simulink model "afe_dq_inv_3L_psm"  (R2025a)
settings: Solver=ode1be  StartTime=0.0  StopTime=simlength  FixedStep=tc  MaxStep=tc
undefined symbols (not defined in the file): Adrso, Amplitude_U, Amplitude_V, Amplitude_W, b, Crso, CTRPIFF_CLIP_RELEASE, dead_time_AFE, dead_time_INV, deepNEGeta, deepNEGxi, deepPOSxi, emf_fb_p, emf_fb_p_ccaller_1, emf_fb_p_ccaller_2, emf_p, emf_p_ccaller_1, emf_p_ccaller_2, end_time_LVRT, fPWM_AFE, fPWM_INV, g0_500Hz, g1_500Hz, ibez, id_lim, Igrid_phase_normalization_factor, iq_lim, ixi_pos_ref_lim, Jm, kg, ki_afe, ki_i, ki_rc_grid, ki_vs, ki_w, kp_afe, kp_i, kp_rc_grid, kp_vs, kp_w, kw, Ld_norm, Ldrso, Lq_norm, Ls_norm, magnitude, motorc_m_scale, n1, n10, omega_bez, omega_grid_emulator_nom, omega_grid_nom, omega_m_bez, omega_m_sim, Phase_shift, pll_i1, pll_i1_ddsrt, pll_p, pll_p_ddsrt, pll_p_frt ... (+28)
libraries: fl_lib x159, nesl_utility x86, cstblocks x14, single_phase_transformer_lib x3, threephase_inductor_lib x2, simulink x2, flexshaft_lib x1, pmsm_uvw_with_harmonics_lib x1
(part 8 of 9)

== system afe_dq_inv_3L_psm/afe_dq_inv_psm_mod1/afe_control/grid_voltage_phase_lock_loops/DQ-PLL/pll_stageA/mormalization_and_transformation ==
  ug_a : Inport
  ug_b : Inport  Port=2
  ug_c : Inport  Port=3
  Gain1 : Gain  Gain=1/Vgrid_phase_normalization_factor
  Gain2 : Gain  Gain=1/Vgrid_phase_normalization_factor
  Gain3 : Gain  Gain=1/Vgrid_phase_normalization_factor
  Mux : Mux  Inputs=3
  Quantizer1 : Quantizer  QuantizationInterval=adc_quantization
  Quantizer2 : Quantizer  QuantizationInterval=adc_quantization
  Quantizer4 : Quantizer  QuantizationInterval=adc_quantization
  Unit Delay : UnitDelay  SampleTime=ts_afe  HasFrameUpgradeWarning=on
  Unit Delay1 : UnitDelay  SampleTime=ts_afe  HasFrameUpgradeWarning=on
  Unit Delay2 : UnitDelay  SampleTime=ts_afe  HasFrameUpgradeWarning=on
  Zero-Order Hold1 : ZeroOrderHold  SampleTime=-1
  Zero-Order Hold3 : ZeroOrderHold  SampleTime=-1
  Zero-Order Hold4 : ZeroOrderHold  SampleTime=-1
  abc2alphabeta : MATLAB Function  TreatAsAtomicUnit=on  SystemSampleTime=ts_afe
  u_500Hz_flt : Subsystem
  u_500Hz_flt1 : Subsystem
  u_500Hz_flt2 : Subsystem
  ug_alpha : Outport  VectorParamsAs1DForOutWhenUnconnected=off
  ug_beta : Outport  Port=2  VectorParamsAs1DForOutWhenUnconnected=off
  tag scope: v_grid_ff_abc=global
  wires:
  abc2alphabeta/2(beta) -> ug_beta/1  "u_grid_beta"
  abc2alphabeta/1(alpha) -> ug_alpha/1  "u_grid_alpha"
  u_500Hz_flt1/1(output) -> Mux/2
  u_500Hz_flt2/1(output) -> Mux/3
  u_500Hz_flt/1(output) -> Mux/1
  Unit Delay/1 -> u_500Hz_flt2/1(input), abc2alphabeta/3(c)
  Unit Delay1/1 -> u_500Hz_flt1/1(input), abc2alphabeta/2(b)
  Mux/1 -> [v_grid_ff_abc]
  Unit Delay2/1 -> u_500Hz_flt/1(input), abc2alphabeta/1(a)
  Zero-Order Hold4/1 -> Unit Delay/1
  Gain1/1 -> Quantizer4/1
  Gain2/1 -> Quantizer1/1
  ug_a/1 -> Gain3/1
  Gain3/1 -> Quantizer2/1
  ug_c/1 -> Gain1/1
  Quantizer2/1 -> Zero-Order Hold1/1
  Zero-Order Hold3/1 -> Unit Delay1/1
  ug_b/1 -> Gain2/1
  Quantizer1/1 -> Zero-Order Hold3/1
  Quantizer4/1 -> Zero-Order Hold4/1
  Zero-Order Hold1/1 -> Unit Delay2/1

== system afe_dq_inv_3L_psm/afe_dq_inv_psm_mod1/afe_control/grid_voltage_phase_lock_loops/DQ-PLL/pll_stageA/sequences ==
  u_grid_alpha : Inport
  u_grid_beta : Inport  Port=2
  gamma_grid : Inport  Port=3
  alphabeta2xieta : Subsystem
  u_grid_pos_xi : Outport
  u_grid_pos_eta : Outport  Port=2
  wires:
  alphabeta2xieta/1(xi) -> u_grid_pos_xi/1  "u_grid_pos_xi"
  alphabeta2xieta/2(eta) -> u_grid_pos_eta/1  "u_grid_pos_eta"
  u_grid_alpha/1 -> alphabeta2xieta/1(alpha)  "u_grid_alpha"
  u_grid_beta/1 -> alphabeta2xieta/2(beta)  "u_grid_beta"
  gamma_grid/1 -> alphabeta2xieta/3(gamma)  "gamma_grid"

== system afe_dq_inv_3L_psm/afe_dq_inv_psm_mod1/afe_control/grid_voltage_phase_lock_loops/DQ-PLL/pll_stageB/double_integrator_observer ==
  theta : Inport
  Gain : Gain  Gain=Ldrso  Multiplication=Matrix(K*u)
  Gain1 : Gain  Gain=Adrso  Multiplication=Matrix(K*u)
  Gain2 : Gain  Gain=Crso  Multiplication=Matrix(K*u)
  Selector : Selector  InputPortWidth=2  IndexOptions=Index vector (dialog)  Indices=2  OutputSizes=1
  Sum : Sum  Inputs=-+|
  Sum1 : Sum  Inputs=|++
  Unit Delay : UnitDelay  SampleTime=ts_afe  HasFrameUpgradeWarning=on
  Zero-Order Hold : ZeroOrderHold  SampleTime=ts_afe
  bounder1 : MATLAB Function  TreatAsAtomicUnit=on  SystemSampleTime=ts_afe
  bounder2 : MATLAB Function  TreatAsAtomicUnit=on  SystemSampleTime=ts_afe
  omega_hat : Outport
  wires:
  Gain/1 -> Sum1/1
  Selector/1 -> omega_hat/1
  Gain2/1 -> bounder2/1(u)  "theta_hat"
  Gain1/1 -> Sum1/2
  Sum1/1 -> Unit Delay/1
  Sum/1 -> bounder1/1(u)  "e"
  Unit Delay/1 -> Gain1/1, Selector/1, Gain2/1
  theta/1 -> Zero-Order Hold/1  "theta"
  Zero-Order Hold/1 -> Sum/2  "theta_dsp"
  bounder1/1(y) -> Gain/1  "e_bounded"
  bounder2/1(y) -> Sum/1  "theta_hat_bounded"

== system afe_dq_inv_3L_psm/afe_dq_inv_psm_mod1/afe_control/grid_voltage_phase_lock_loops/DQ-PLL/pll_stageB/scheduled-p-gain ==
  In1 : Inport
  Switch : Switch  Criteria=u2 > Threshold  Threshold=0.5  SaturateOnIntegerOverflow=off  InputSameDT=off
  kp1 : Gain  Gain=pll_p  SaturateOnIntegerOverflow=on  OutDataTypeStr=Inherit: Same as input  ParamDataTypeStr=Inherit: Same as input
  kp3 : Gain  Gain=pll_p_frt  SaturateOnIntegerOverflow=on  OutDataTypeStr=Inherit: Same as input  ParamDataTypeStr=Inherit: Same as input
  Out2 : Outport
  wires:
  kp3/1 -> Switch/1
  kp1/1 -> Switch/3
  [frt_active] -> Switch/2
  In1/1 -> kp1/1, kp3/1
  Switch/1 -> Out2/1

== system afe_dq_inv_3L_psm/afe_dq_inv_psm_mod1/inverter/inverter/sv_pwm/modulator1/PWM generator u ==
  m : Inport
  phase : Inport  Port=2
  Bus Creator : BusCreator  Inputs=4
  Constant : Constant
  Gain : Gain  Gain=2
  Sum : Sum  Inputs=|+-
  carry_p : Subsystem
  modulator_n1 : Subsystem
  modulator_p1 : Subsystem
  mu : Outport
  wires:
  phase/1 -> carry_p/1(phase)
  carry_p/1(trp) -> modulator_n1/1(tr), modulator_p1/1(tr)  "trp"
  modulator_p1/1(m1) -> [m1]
  modulator_p1/2(m3) -> [m3]
  modulator_n1/1(m2) -> [m2]
  modulator_n1/2(m4) -> [m4]
  [m1] -> Bus Creator/1  "m1u"
  [m2] -> Bus Creator/2  "m2u"
  [m3] -> Bus Creator/3  "m3u"
  [m4] -> Bus Creator/4  "m4u"
  Bus Creator/1 -> mu/1  "p"
  m/1 -> Gain/1
  Gain/1 -> Sum/1
  Constant/1 -> Sum/2
  Sum/1 -> modulator_p1/2(m_index), modulator_n1/2(m_index)

== system afe_dq_inv_3L_psm/afe_dq_inv_psm_mod1/inverter/inverter/sv_pwm/modulator1/PWM generator v ==
  m : Inport
  phase : Inport  Port=2
  Bus Creator : BusCreator  Inputs=4
  Constant : Constant
  Gain : Gain  Gain=2
  Sum : Sum  Inputs=|+-
  carry_p : Subsystem
  modulator_n1 : Subsystem
  modulator_p1 : Subsystem
  mv : Outport
  wires:
  Sum/1 -> modulator_n1/2(m_index), modulator_p1/2(m_index)
  Constant/1 -> Sum/2
  Gain/1 -> Sum/1
  m/1 -> Gain/1
  Bus Creator/1 -> mv/1  "p"
  [m4] -> Bus Creator/4  "m4v"
  [m3] -> Bus Creator/3  "m3v"
  [m2] -> Bus Creator/2  "m2v"
  [m1] -> Bus Creator/1  "m1v"
  modulator_n1/2(m4) -> [m4]
  modulator_n1/1(m2) -> [m2]
  modulator_p1/2(m3) -> [m3]
  modulator_p1/1(m1) -> [m1]
  carry_p/1(trp) -> modulator_p1/1(tr), modulator_n1/1(tr)  "trp"
  phase/1 -> carry_p/1(phase)

== system afe_dq_inv_3L_psm/afe_dq_inv_psm_mod1/inverter/inverter/sv_pwm/modulator1/PWM generator w ==
  m : Inport
  phase : Inport  Port=2
  Bus Creator : BusCreator  Inputs=4
  Constant : Constant
  Gain : Gain  Gain=2
  Sum : Sum  Inputs=|+-
  carry_p : Subsystem
  modulator_n1 : Subsystem
  modulator_p1 : Subsystem
  mw : Outport
  wires:
  phase/1 -> carry_p/1(phase)
  carry_p/1(trp) -> modulator_n1/1(tr), modulator_p1/1(tr)  "trp"
  modulator_p1/1(m1) -> [m1]
  modulator_p1/2(m3) -> [m3]
  modulator_n1/1(m2) -> [m2]
  modulator_n1/2(m4) -> [m4]
  [m1] -> Bus Creator/1  "m1w"
  [m2] -> Bus Creator/2  "m2w"
  [m3] -> Bus Creator/3  "m3w"
  [m4] -> Bus Creator/4  "m4w"
  Bus Creator/1 -> mw/1  "p"
  m/1 -> Gain/1
  Gain/1 -> Sum/1
  Constant/1 -> Sum/2
  Sum/1 -> modulator_p1/2(m_index), modulator_n1/2(m_index)

== system afe_dq_inv_3L_psm/afe_dq_inv_psm_mod1/inverter_control/current_ctrl/bemf_observer/bemf_observer/double_integrator_observer ==
  theta : Inport
  Dead Zone : DeadZone  LowerValue=-0.01  UpperValue=0.01
  Gain : Gain  Gain=kw
  Gain1 : Gain  Gain=kg
  Gain2 : Gain  Gain=omega_bez
  Gain3 : Gain  Gain=1/omega_bez
  Gain5 : Gain  Gain=ts_inv
  Sum : Sum  Inputs=-+|
  Sum1 : Sum  Inputs=|++
  Sum2 : Sum  Inputs=|++
  Sum8 : Sum  Inputs=++|
  Unit Delay1 : UnitDelay  InitialCondition=pi  SampleTime=ts_inv  HasFrameUpgradeWarning=on
  Unit Delay2 : UnitDelay  SampleTime=ts_inv  HasFrameUpgradeWarning=on
  bounder1 : MATLAB Function  TreatAsAtomicUnit=on  SystemSampleTime=ts_inv
  bounder2 : MATLAB Function  TreatAsAtomicUnit=on  SystemSampleTime=ts_inv
  omega_pu_hat : Outport  VectorParamsAs1DForOutWhenUnconnected=off
  theta_hat : Outport  Port=2  VectorParamsAs1DForOutWhenUnconnected=off
  wires:
  Gain1/1 -> Sum2/1
  theta/1 -> Sum/2  "theta_bemf"
  Sum8/1 -> Unit Delay1/1
  Unit Delay1/1 -> bounder2/1(u)
  Sum1/1 -> Unit Delay2/1
  Gain/1 -> Gain3/1
  Unit Delay2/1 -> omega_pu_hat/1, Sum1/2, Gain5/1
  Sum2/1 -> Sum8/2
  bounder2/1(y) -> Sum2/2, theta_hat/1, Sum/1  "theta_hat"
  bounder1/1(y) -> Gain1/1, Gain/1
  Gain2/1 -> Sum8/1
  Gain3/1 -> Sum1/1
  Gain5/1 -> Gain2/1
  Sum/1 -> bounder1/1(u)

== system afe_dq_inv_3L_psm/afe_dq_inv_psm_mod1/inverter_control/current_ctrl/bemf_observer/bemf_observer/psi_alpha_hat ==
  ualpha : Inport
  ialpha : Inport  Port=2
  Gain1 : Gain  Gain=Rs_norm
  Gain2 : Gain  Gain=emf_fb_p
  Gain3 : Gain  Gain=emf_p
  Gain4 : Gain  Gain=omega_bez
  Gain5 : Gain  Gain=Ls_norm
  Gain6 : Gain  Gain=motorc_m_scale
  Gain7 : Gain  Gain=ts_inv
  Product : Product  RndMeth=Zero
  Sum : Sum  Inputs=|+-
  Sum1 : Sum  Inputs=|+-
  Sum2 : Sum  Inputs=++-  SaturateOnIntegerOverflow=on
  Sum3 : Sum  Inputs=|++
  Sum4 : Sum  Inputs=+-  SaturateOnIntegerOverflow=on
  Unit Delay1 : UnitDelay  SampleTime=ts_inv  HasFrameUpgradeWarning=on
  Unit Delay2 : UnitDelay  SampleTime=ts_inv  HasFrameUpgradeWarning=on
  Unit Delay3 : UnitDelay  SampleTime=ts_inv  HasFrameUpgradeWarning=on
  psi_s_alpha_hat : Outport  VectorParamsAs1DForOutWhenUnconnected=off
  psi_r_alpha_hat : Outport  Port=2  VectorParamsAs1DForOutWhenUnconnected=off
  wires:
  [psi_r_m_alpha] -> Sum1/1
  [psi_r_alpha_hat] -> Sum1/2
  Gain4/1 -> Gain7/1
  Sum2/1 -> Gain4/1
  Gain3/1 -> Sum2/3
  ialpha/1 -> Gain5/1, Gain1/1
  Gain1/1 -> Sum/2
  Sum/1 -> Sum2/2
  ualpha/1 -> Product/1
  Gain5/1 -> Unit Delay3/1
  Unit Delay1/1 -> Sum4/1, psi_s_alpha_hat/1, Gain3/1, Sum3/2
  Sum3/1 -> Unit Delay1/1
  Sum4/1 -> Unit Delay2/1
  Sum1/1 -> Gain2/1
  Gain2/1 -> Sum2/1
  [vdc_pu] -> Product/2
  Gain7/1 -> Sum3/1
  Product/1 -> Gain6/1
  Gain6/1 -> Sum/1
  Unit Delay2/1 -> psi_r_alpha_hat/1
  Unit Delay3/1 -> Sum4/2

== system afe_dq_inv_3L_psm/afe_dq_inv_psm_mod1/inverter_control/current_ctrl/bemf_observer/bemf_observer/psi_beta_hat ==
  ubeta : Inport
  ibeta : Inport  Port=2
  Gain1 : Gain  Gain=Rs_norm
  Gain2 : Gain  Gain=emf_fb_p
  Gain3 : Gain  Gain=emf_p
  Gain4 : Gain  Gain=omega_bez
  Gain5 : Gain  Gain=Ls_norm
  Gain6 : Gain  Gain=motorc_m_scale
  Gain7 : Gain  Gain=ts_inv
  Product : Product  RndMeth=Zero
  Sum : Sum  Inputs=|+-
  Sum1 : Sum  Inputs=|+-
  Sum2 : Sum  Inputs=++-  SaturateOnIntegerOverflow=on
  Sum3 : Sum  Inputs=|++
  Sum4 : Sum  Inputs=+-  SaturateOnIntegerOverflow=on
  Unit Delay1 : UnitDelay  SampleTime=ts_inv  HasFrameUpgradeWarning=on
  Unit Delay2 : UnitDelay  SampleTime=ts_inv  HasFrameUpgradeWarning=on
  Unit Delay3 : UnitDelay  SampleTime=ts_inv  HasFrameUpgradeWarning=on
  psi_s_beta_hat : Outport  VectorParamsAs1DForOutWhenUnconnected=off
  psi_r_beta_hat : Outport  Port=2  VectorParamsAs1DForOutWhenUnconnected=off
  wires:
  Gain5/1 -> Unit Delay3/1
  Sum/1 -> Sum2/2
  Gain1/1 -> Sum/2
  ibeta/1 -> Gain5/1, Gain1/1
  Gain3/1 -> Sum2/3
  Sum2/1 -> Gain4/1
  Gain4/1 -> Gain7/1
  Sum1/1 -> Gain2/1
  [psi_r_beta_hat] -> Sum1/2
  [psi_r_m_beta] -> Sum1/1
  Unit Delay1/1 -> Gain3/1, Sum4/1, psi_s_beta_hat/1, Sum3/2
  Sum3/1 -> Unit Delay1/1
  Sum4/1 -> Unit Delay2/1
  Gain2/1 -> Sum2/1
  ubeta/1 -> Product/1
  [vdc_pu] -> Product/2
  Gain7/1 -> Sum3/1
  Product/1 -> Gain6/1
  Gain6/1 -> Sum/1
  Unit Delay2/1 -> psi_r_beta_hat/1
  Unit Delay3/1 -> Sum4/2

== system afe_dq_inv_3L_psm/afe_dq_inv_psm_mod1/inverter_control/current_ctrl/bemf_observer/bemf_observer/theta_bemf_hat ==
  psi_r_alpha_hat : Inport
  psi_r_beta_hat : Inport  Port=2
  Trigonometric Function : Trigonometry  Operator=atan2  OutputSignalType=real
  theta_emf_hat : Outport  VectorParamsAs1DForOutWhenUnconnected=off
  wires:
  psi_r_alpha_hat/1 -> Trigonometric Function/2
  psi_r_beta_hat/1 -> Trigonometric Function/1
  Trigonometric Function/1 -> theta_emf_hat/1

== system afe_dq_inv_3L_psm/afe_dq_inv_psm_mod1/inverter_control/current_ctrl/bemf_observer/bemf_observer_ccaller/Reset Trigger ==
  Step : Step  Time=0.01  Before=1  After=0  SampleTime=0
  Out1 : Outport
  wires:
  Step/1 -> Out1/1  "Reset"

== system afe_dq_inv_3L_psm/afe_dq_inv_psm_mod1/inverter_control/current_ctrl/bemf_observer/phase_fault/drop_phase_zerofor_delta_time ==
  theta_pmsm : Inport
  Product : Product
  Step : Step  Time=time_phase_fault  Before=1  After=0  SampleTime=0
  Step1 : Step  Time=time_phase_fault+3e-3  SampleTime=0
  Sum : Sum  Inputs=|++
  theta : Outport
  wires:
  theta_pmsm/1 -> Product/1
  Step1/1 -> Sum/2
  Product/1 -> theta/1
  Sum/1 -> Product/2
  Step/1 -> Sum/1

== system afe_dq_inv_3L_psm/afe_dq_inv_psm_mod1/inverter_control/current_ctrl/bemf_observer/phase_fault/hold_phase_for_delta_time ==
  theta_pmsm : Inport
  Enabled Subsystem : Subsystem  TreatAsAtomicUnit=on
  Step : Step  Time=time_phase_fault  Before=1  After=0  SampleTime=0
  Step1 : Step  Time=time_phase_fault+25e-3  SampleTime=0
  Sum : Sum  Inputs=|++
  theta : Outport
  wires:
  Step/1 -> Sum/1
  Step1/1 -> Sum/2
  theta_pmsm/1 -> Enabled Subsystem/1(theta_pmsm)
  Enabled Subsystem/1(theta) -> theta/1
  Sum/1 -> Enabled Subsystem/Enable

== system afe_dq_inv_3L_psm/afe_dq_inv_psm_mod1/inverter_control/current_ctrl/bemf_observer/phase_fault/loss_phase ==
  theta_pmsm : Inport
  Enabled Subsystem : Subsystem  TreatAsAtomicUnit=on
  Step : Step  Time=time_phase_fault  Before=1  After=0  SampleTime=0
  theta : Outport
  wires:
  Step/1 -> Enabled Subsystem/Enable
  Enabled Subsystem/1(theta) -> theta/1
  theta_pmsm/1 -> Enabled Subsystem/1(theta_pmsm)

== system afe_dq_inv_3L_psm/afe_dq_inv_psm_mod1/inverter_control/current_ctrl/current_ctrl/dq_pi_with_vector_antiwindup/dq_vector_pi ==
  id : Inport
  id_ref : Inport  Port=2
  iq : Inport  Port=3
  iq_ref : Inport  Port=4
  Sum1 : Sum  Inputs=|-+
  Sum2 : Sum  Inputs=|-+
  bounder1 : Subsystem
  bounder2 : Subsystem
  pi_d : Subsystem
  pi_q : Subsystem
  switch : Subsystem
  vector lenght : Subsystem
  md_sat : Outport
  mq_sat : Outport  Port=2
  wires:
  bounder2/2(clip) -> switch/2(clip 2)
  vector lenght/2(m) -> bounder1/3(m), bounder2/1(m)
  Sum2/1 -> pi_q/1(iq_tilde)
  pi_d/1(ud_out) -> vector lenght/1(md), bounder1/1(md)
  pi_q/1(Vqs_out) -> bounder2/3(mq), vector lenght/2(mq)
  vector lenght/1(m_1) -> bounder1/2(m_1), bounder2/2(m_1)
  switch/1(clip) -> pi_q/2(clip), pi_d/2(clip)
  iq/1 -> Sum2/1
  Sum1/1 -> pi_d/1(id_tilde)
  bounder1/2(clip) -> switch/1(clip 1)
  id/1 -> Sum1/1
  bounder1/1(md_sat) -> md_sat/1
  bounder2/1(mq_sat) -> mq_sat/1
  id_ref/1 -> Sum1/2
  iq_ref/1 -> Sum2/2

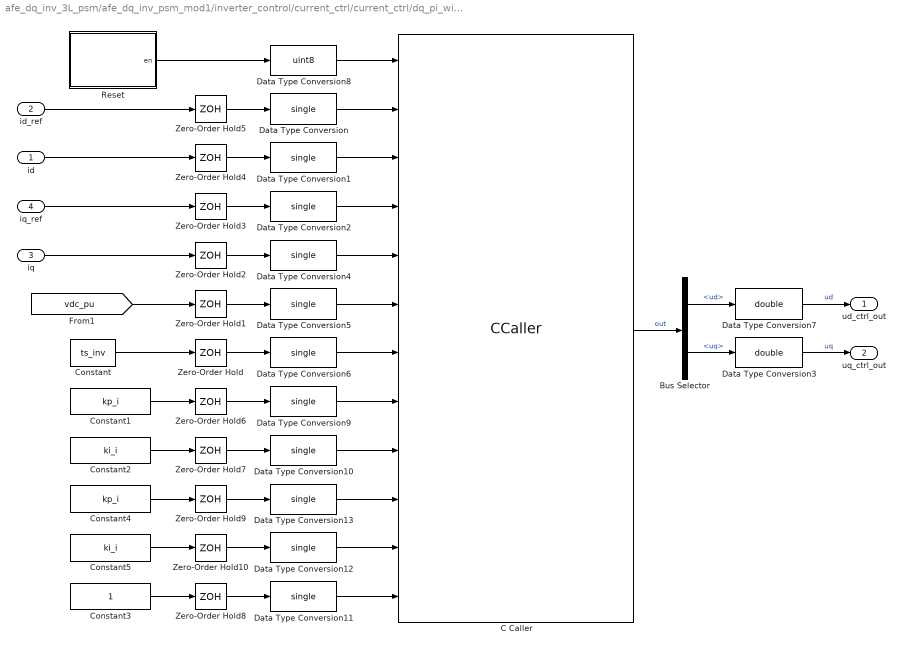
== system afe_dq_inv_3L_psm/afe_dq_inv_psm_mod1/inverter_control/current_ctrl/current_ctrl/dq_pi_with_vector_antiwindup/dq_vector_pi_ccaller ==
  id : Inport
  id_ref : Inport  Port=2
  iq : Inport  Port=3
  iq_ref : Inport  Port=4
  Bus Selector : BusSelector  OutputSignals=ud,uq
  C Caller : CCaller  FunctionName=dqvector_pi_process_simulink  PortSpecificationStruct="%)30     .    ,!8   8    (     @         %    \"     T    !     0         %  0 \"0    $    _    07)G3F%M90  4&]R=$YA;64 4V-O<&4     26YD97@     5'EP90      4VEZ90      27-';&]B86P   X    P    !@    @    $          4    (     0    ,    !         !   P!O=70 #@   #     &    \"     0         !0    @    !     P    $         $  # &]U=  .    .     8    (    !          %    \"     $    &     0         0   ...(+7280 chars)"  SampleTime=ts_inv
  Constant : Constant  Value=ts_inv
  Constant1 : Constant  Value=kp_i
  Constant2 : Constant  Value=ki_i
  Constant3 : Constant
  Constant4 : Constant  Value=kp_i
  Constant5 : Constant  Value=ki_i
  Data Type Conversion{,1..2,4..6,9..13} (11 alike) : DataTypeConversion  OutDataTypeStr=single  SaturateOnIntegerOverflow=off  RndMeth=Floor
  Data Type Conversion3 : DataTypeConversion  OutDataTypeStr=double  SaturateOnIntegerOverflow=off  RndMeth=Floor
  Data Type Conversion7 : DataTypeConversion  OutDataTypeStr=double  SaturateOnIntegerOverflow=off  RndMeth=Floor
  Data Type Conversion8 : DataTypeConversion  OutDataTypeStr=uint8  SaturateOnIntegerOverflow=off  RndMeth=Floor
  Reset : Subsystem
  Zero-Order Hold{,1..10} (11 alike) : ZeroOrderHold  SampleTime=ts_inv
  ud_ctrl_out : Outport
  uq_ctrl_out : Outport  Port=2
  wires:
  Data Type Conversion5/1 -> C Caller/6
  Data Type Conversion/1 -> C Caller/2
  C Caller/1 -> Bus Selector/1  "out"
  Data Type Conversion1/1 -> C Caller/3
  Data Type Conversion4/1 -> C Caller/5
  Data Type Conversion2/1 -> C Caller/4
  Data Type Conversion6/1 -> C Caller/7
  Zero-Order Hold/1 -> Data Type Conversion6/1
  Zero-Order Hold5/1 -> Data Type Conversion/1
  Zero-Order Hold4/1 -> Data Type Conversion1/1
  Zero-Order Hold3/1 -> Data Type Conversion2/1
  Zero-Order Hold2/1 -> Data Type Conversion4/1
  Zero-Order Hold1/1 -> Data Type Conversion5/1
  [vdc_pu] -> Zero-Order Hold1/1
  Constant/1 -> Zero-Order Hold/1
  id_ref/1 -> Zero-Order Hold5/1
  iq_ref/1 -> Zero-Order Hold3/1
  id/1 -> Zero-Order Hold4/1
  iq/1 -> Zero-Order Hold2/1
  Bus Selector/2 -> Data Type Conversion3/1  "<uq>"
  Bus Selector/1 -> Data Type Conversion7/1  "<ud>"
  Data Type Conversion7/1 -> ud_ctrl_out/1  "ud"
  Data Type Conversion3/1 -> uq_ctrl_out/1  "uq"
  Reset/1(en) -> Data Type Conversion8/1
  Data Type Conversion8/1 -> C Caller/1
  Constant1/1 -> Zero-Order Hold6/1
  Zero-Order Hold6/1 -> Data Type Conversion9/1
  Data Type Conversion9/1 -> C Caller/8
  Data Type Conversion10/1 -> C Caller/9
  Zero-Order Hold7/1 -> Data Type Conversion10/1
  Zero-Order Hold8/1 -> Data Type Conversion11/1
  Constant2/1 -> Zero-Order Hold7/1
  Constant3/1 -> Zero-Order Hold8/1
  Data Type Conversion11/1 -> C Caller/12
  Constant5/1 -> Zero-Order Hold10/1
  Zero-Order Hold10/1 -> Data Type Conversion12/1
  Zero-Order Hold9/1 -> Data Type Conversion13/1
  Constant4/1 -> Zero-Order Hold9/1
  Data Type Conversion13/1 -> C Caller/10
  Data Type Conversion12/1 -> C Caller/11

== system afe_dq_inv_3L_psm/afe_dq_inv_psm_mod1/afe_control/grid_voltage_phase_lock_loops/DDSRF-PLL/pll_stageA/sequences/ddsrf ==
  u_grid_alpha : Inport
  u_grid_beta : Inport  Port=2
  phase_angle : Inport  Port=3
  Gain : Gain  Gain=2
  LTI System{,1..3} (4 alike) : cstblocks/LTI System  sys=ddsrf_fd  IC=[]  PadeOrder=0
  Sum : Sum  Inputs=|+-
  Sum1 : Sum  Inputs=|+-
  Sum2 : Sum  Inputs=-+|
  Sum3 : Sum  Inputs=-+|
  alphabeta2xieta_neg : MATLAB Function  TreatAsAtomicUnit=on
  alphabeta2xieta_neg1 : MATLAB Function  TreatAsAtomicUnit=on
  alphabeta2xieta_pos : MATLAB Function  TreatAsAtomicUnit=on
  alphabeta2xieta_pos1 : MATLAB Function  TreatAsAtomicUnit=on
  bounder2 : MATLAB Function  TreatAsAtomicUnit=on  SystemSampleTime=ts_afe
  u_grid_pos_xi : Outport
  u_grid_pos_eta : Outport  Port=2
  u_grid_neg_xi : Outport  Port=3
  u_grid_neg_eta : Outport  Port=4
  wires:
  phase_angle/1 -> alphabeta2xieta_pos/3(gamma), alphabeta2xieta_neg/3(gamma), Gain/1  "phase_angle"
  u_grid_beta/1 -> alphabeta2xieta_pos/2(beta), alphabeta2xieta_neg/2(beta)  "u_grid_beta"
  u_grid_alpha/1 -> alphabeta2xieta_pos/1(alpha), alphabeta2xieta_neg/1(alpha)  "u_grid_alpha"
  alphabeta2xieta_pos/1(xi) -> Sum/1  "u_grid_pos_xi"
  Sum/1 -> LTI System/1
  alphabeta2xieta_pos/2(eta) -> Sum1/1  "u_grid_pos_eta"
  Sum1/1 -> LTI System1/1
  alphabeta2xieta_neg/1(xi) -> Sum2/2  "u_grid_neg_xi"
  Sum2/1 -> LTI System2/1
  Sum3/1 -> LTI System3/1
  alphabeta2xieta_neg/2(eta) -> Sum3/2  "u_grid_neg_eta"
  Gain/1 -> bounder2/1(u)
  LTI System/1 -> alphabeta2xieta_neg1/1(alpha), u_grid_pos_xi/1
  LTI System1/1 -> alphabeta2xieta_neg1/2(beta), u_grid_pos_eta/1
  LTI System2/1 -> u_grid_neg_xi/1, alphabeta2xieta_pos1/1(alpha)
  LTI System3/1 -> u_grid_neg_eta/1, alphabeta2xieta_pos1/2(beta)
  bounder2/1(y) -> [phase_angle_2]
  [phase_angle_2] -> alphabeta2xieta_pos1/3(gamma)
  [phase_angle_2] -> alphabeta2xieta_neg1/3(gamma)
  alphabeta2xieta_pos1/1(xi) -> Sum/2
  alphabeta2xieta_pos1/2(eta) -> Sum1/2
  alphabeta2xieta_neg1/1(xi) -> Sum2/1
  alphabeta2xieta_neg1/2(eta) -> Sum3/1

== system afe_dq_inv_3L_psm/afe_dq_inv_psm_mod1/afe_control/grid_voltage_phase_lock_loops/DQ-PLL/pll_stageA/mormalization_and_transformation/u_500Hz_flt ==
  input : Inport
  Gain3 : Gain  Gain=g1_500Hz
  Gain6 : Gain  Gain=g0_500Hz
  Sum : Sum  Inputs=|++
  Unit Delay1 : UnitDelay  SampleTime=ts_afe  HasFrameUpgradeWarning=on
  output : Outport  VectorParamsAs1DForOutWhenUnconnected=off
  wires:
  Sum/1 -> output/1, Unit Delay1/1
  Gain3/1 -> Sum/2
  Unit Delay1/1 -> Gain3/1
  input/1 -> Gain6/1
  Gain6/1 -> Sum/1

== system afe_dq_inv_3L_psm/afe_dq_inv_psm_mod1/afe_control/grid_voltage_phase_lock_loops/DQ-PLL/pll_stageA/mormalization_and_transformation/u_500Hz_flt1 ==
  input : Inport
  Gain3 : Gain  Gain=g1_500Hz
  Gain6 : Gain  Gain=g0_500Hz
  Sum : Sum  Inputs=|++
  Unit Delay1 : UnitDelay  SampleTime=ts_afe  HasFrameUpgradeWarning=on
  output : Outport  VectorParamsAs1DForOutWhenUnconnected=off
  wires:
  Gain6/1 -> Sum/1
  input/1 -> Gain6/1
  Unit Delay1/1 -> Gain3/1
  Gain3/1 -> Sum/2
  Sum/1 -> Unit Delay1/1, output/1

== system afe_dq_inv_3L_psm/afe_dq_inv_psm_mod1/afe_control/grid_voltage_phase_lock_loops/DQ-PLL/pll_stageA/mormalization_and_transformation/u_500Hz_flt2 ==
  input : Inport
  Gain3 : Gain  Gain=g1_500Hz
  Gain6 : Gain  Gain=g0_500Hz
  Sum : Sum  Inputs=|++
  Unit Delay1 : UnitDelay  SampleTime=ts_afe  HasFrameUpgradeWarning=on
  output : Outport  VectorParamsAs1DForOutWhenUnconnected=off
  wires:
  Sum/1 -> output/1, Unit Delay1/1
  Gain3/1 -> Sum/2
  Unit Delay1/1 -> Gain3/1
  input/1 -> Gain6/1
  Gain6/1 -> Sum/1

== system afe_dq_inv_3L_psm/afe_dq_inv_psm_mod1/afe_control/grid_voltage_phase_lock_loops/DQ-PLL/pll_stageA/sequences/alphabeta2xieta ==
  alpha : Inport
  beta : Inport  Port=2
  gamma : Inport  Port=3
  alphabeta2xieta_neg : MATLAB Function  TreatAsAtomicUnit=on  SystemSampleTime=ts_afe
  alphabeta2xieta_pos : MATLAB Function  TreatAsAtomicUnit=on  SystemSampleTime=ts_afe
  xi : Outport
  eta : Outport  Port=2
  Out3 : Outport  Port=3
  Out4 : Outport  Port=4
  wires:
  alpha/1 -> alphabeta2xieta_neg/1(alpha), alphabeta2xieta_pos/1(alpha)  "u_grid_alpha"
  beta/1 -> alphabeta2xieta_neg/2(beta), alphabeta2xieta_pos/2(beta)  "u_grid_beta"
  gamma/1 -> alphabeta2xieta_neg/3(gamma), alphabeta2xieta_pos/3(gamma)  "gamma_grid"
  alphabeta2xieta_pos/1(xi) -> xi/1  "u_grid_pos_xi"
  alphabeta2xieta_pos/2(eta) -> eta/1  "u_grid_pos_eta"
  alphabeta2xieta_neg/1(xi) -> Out3/1  "u_grid_neg_xi"
  alphabeta2xieta_neg/2(eta) -> Out4/1  "u_grid_neg_eta"

== system afe_dq_inv_3L_psm/afe_dq_inv_psm_mod1/inverter/inverter/sv_pwm/modulator1/PWM generator u/carry_p ==
  phase : Inport
  Clock : Clock
  Constant2 : Constant  Value=1/f
  Constant4 : Constant
  Gain4 : Gain  Gain=1/2
  Gain5 : Gain  Gain=1/(pi/2)
  MATLAB Function : MATLAB Function  TreatAsAtomicUnit=on
  Sum3 : Sum  Inputs=|++
  trp : Outport
  wires:
  Gain5/1 -> Sum3/1
  Gain4/1 -> trp/1
  Constant2/1 -> MATLAB Function/3(period)
  Sum3/1 -> Gain4/1
  MATLAB Function/1(y) -> Gain5/1
  Constant4/1 -> Sum3/2
  Clock/1 -> MATLAB Function/1(t)
  phase/1 -> MATLAB Function/2(phase)

== system afe_dq_inv_3L_psm/afe_dq_inv_psm_mod1/inverter/inverter/sv_pwm/modulator1/PWM generator u/modulator_n1 ==
  tr : Inport
  m_index : Inport  Port=2
  Constant : Constant  Value=dead_time*f
  Constant1 : Constant  Value=polarity
  Constant2 : Constant
  Data Type Conversion1 : DataTypeConversion  OutDataTypeStr=double
  Data Type Conversion2 : DataTypeConversion  OutDataTypeStr=double
  Hit Crossing : HitCross  ShowOutputPort=off
  Hit Crossing1 : HitCross  ShowOutputPort=off
  Relational Operator1 : RelationalOperator  Operator=<  InputSameDT=off
  Relational Operator2 : RelationalOperator  Operator=<=  InputSameDT=off
  Relay : Relay  OnOutputValue=pos_cmd_gate  OffOutputValue=neg_cmd_gate
  Relay1 : Relay  OnOutputValue=pos_cmd_gate  OffOutputValue=neg_cmd_gate
  Saturation1 : Saturate  UpperLimit=0  LowerLimit=m_low
  Sum : Sum  Inputs=|++  SaturateOnIntegerOverflow=on
  Sum1 : Sum  Inputs=-+|  SaturateOnIntegerOverflow=on
  Sum2 : Sum  Inputs=++|  SaturateOnIntegerOverflow=on
  Switch : Switch  Criteria=u2 > Threshold  SaturateOnIntegerOverflow=off  InputSameDT=off
  Switch1 : Switch  Criteria=u2 > Threshold  SaturateOnIntegerOverflow=off  InputSameDT=off
  m2 : Outport
  m4 : Outport  Port=2
  wires:
  Relay1/1 -> m4/1
  Relay/1 -> m2/1
  Switch1/1 -> Relay1/1
  tr/1 -> Relational Operator1/2, Relational Operator2/1
  Sum/1 -> Relational Operator1/1
  Constant/1 -> Sum1/1, Sum/2
  Switch/1 -> Relay/1
  Data Type Conversion2/1 -> Hit Crossing1/1, Switch1/3, Switch/1
  Constant1/1 -> Switch/2, Switch1/2
  Sum1/1 -> Relational Operator2/2
  Data Type Conversion1/1 -> Switch1/1, Switch/3, Hit Crossing/1
  Relational Operator1/1 -> Data Type Conversion1/1
  Relational Operator2/1 -> Data Type Conversion2/1
  m_index/1 -> Saturation1/1
  Saturation1/1 -> Sum2/2
  Sum2/1 -> Sum1/2, Sum/1
  Constant2/1 -> Sum2/1

== system afe_dq_inv_3L_psm/afe_dq_inv_psm_mod1/inverter/inverter/sv_pwm/modulator1/PWM generator u/modulator_p1 ==
  tr : Inport
  m_index : Inport  Port=2
  Constant : Constant  Value=dead_time*f
  Constant1 : Constant  Value=polarity
  Data Type Conversion1 : DataTypeConversion  OutDataTypeStr=double
  Data Type Conversion2 : DataTypeConversion  OutDataTypeStr=double
  Hit Crossing : HitCross  ShowOutputPort=off
  Hit Crossing1 : HitCross  ShowOutputPort=off
  Relational Operator1 : RelationalOperator  Operator=<  InputSameDT=off
  Relational Operator2 : RelationalOperator  Operator=<  InputSameDT=off
  Relay : Relay  OnSwitchValue=2*eps  OnOutputValue=pos_cmd_gate  OffOutputValue=neg_cmd_gate
  Relay1 : Relay  OnOutputValue=pos_cmd_gate  OffOutputValue=neg_cmd_gate
  Saturation1 : Saturate  UpperLimit=m_up  LowerLimit=0
  Sum : Sum  Inputs=|++  SaturateOnIntegerOverflow=on
  Sum1 : Sum  Inputs=-+|  SaturateOnIntegerOverflow=on
  Switch : Switch  Criteria=u2 > Threshold  SaturateOnIntegerOverflow=off  InputSameDT=off
  Switch1 : Switch  Criteria=u2 > Threshold  SaturateOnIntegerOverflow=off  InputSameDT=off
  m1 : Outport
  m3 : Outport  Port=2
  wires:
  m_index/1 -> Saturation1/1
  Relational Operator2/1 -> Data Type Conversion2/1
  Relational Operator1/1 -> Data Type Conversion1/1
  Data Type Conversion1/1 -> Hit Crossing/1, Switch/3, Switch1/1
  Sum1/1 -> Relational Operator2/2
  Saturation1/1 -> Sum/1, Sum1/2
  Constant1/1 -> Switch1/2, Switch/2
  Data Type Conversion2/1 -> Switch/1, Switch1/3, Hit Crossing1/1
  Switch/1 -> Relay/1
  Constant/1 -> Sum/2, Sum1/1
  Sum/1 -> Relational Operator1/1
  tr/1 -> Relational Operator2/1, Relational Operator1/2
  Switch1/1 -> Relay1/1
  Relay/1 -> m1/1
  Relay1/1 -> m3/1

== system afe_dq_inv_3L_psm/afe_dq_inv_psm_mod1/inverter/inverter/sv_pwm/modulator1/PWM generator v/carry_p ==
  phase : Inport
  Clock : Clock
  Constant2 : Constant  Value=1/f
  Constant4 : Constant
  Gain4 : Gain  Gain=1/2
  Gain5 : Gain  Gain=1/(pi/2)
  MATLAB Function : MATLAB Function  TreatAsAtomicUnit=on
  Sum3 : Sum  Inputs=|++
  trp : Outport
  wires:
  phase/1 -> MATLAB Function/2(phase)
  Clock/1 -> MATLAB Function/1(t)
  Constant4/1 -> Sum3/2
  MATLAB Function/1(y) -> Gain5/1
  Sum3/1 -> Gain4/1
  Constant2/1 -> MATLAB Function/3(period)
  Gain4/1 -> trp/1
  Gain5/1 -> Sum3/1

== system afe_dq_inv_3L_psm/afe_dq_inv_psm_mod1/inverter/inverter/sv_pwm/modulator1/PWM generator v/modulator_n1 ==
  tr : Inport
  m_index : Inport  Port=2
  Constant : Constant  Value=dead_time*f
  Constant1 : Constant  Value=polarity
  Constant2 : Constant
  Data Type Conversion1 : DataTypeConversion  OutDataTypeStr=double
  Data Type Conversion2 : DataTypeConversion  OutDataTypeStr=double
  Hit Crossing : HitCross  ShowOutputPort=off
  Hit Crossing1 : HitCross  ShowOutputPort=off
  Relational Operator1 : RelationalOperator  Operator=<  InputSameDT=off
  Relational Operator2 : RelationalOperator  Operator=<=  InputSameDT=off
  Relay : Relay  OnOutputValue=pos_cmd_gate  OffOutputValue=neg_cmd_gate
  Relay1 : Relay  OnOutputValue=pos_cmd_gate  OffOutputValue=neg_cmd_gate
  Saturation1 : Saturate  UpperLimit=0  LowerLimit=m_low
  Sum : Sum  Inputs=|++  SaturateOnIntegerOverflow=on
  Sum1 : Sum  Inputs=-+|  SaturateOnIntegerOverflow=on
  Sum2 : Sum  Inputs=++|  SaturateOnIntegerOverflow=on
  Switch : Switch  Criteria=u2 > Threshold  SaturateOnIntegerOverflow=off  InputSameDT=off
  Switch1 : Switch  Criteria=u2 > Threshold  SaturateOnIntegerOverflow=off  InputSameDT=off
  m2 : Outport
  m4 : Outport  Port=2
  wires:
  Constant2/1 -> Sum2/1
  Sum2/1 -> Sum/1, Sum1/2
  Saturation1/1 -> Sum2/2
  m_index/1 -> Saturation1/1
  Relational Operator2/1 -> Data Type Conversion2/1
  Relational Operator1/1 -> Data Type Conversion1/1
  Data Type Conversion1/1 -> Hit Crossing/1, Switch/3, Switch1/1
  Sum1/1 -> Relational Operator2/2
  Constant1/1 -> Switch1/2, Switch/2
  Data Type Conversion2/1 -> Switch/1, Switch1/3, Hit Crossing1/1
  Switch/1 -> Relay/1
  Constant/1 -> Sum/2, Sum1/1
  Sum/1 -> Relational Operator1/1
  tr/1 -> Relational Operator2/1, Relational Operator1/2
  Switch1/1 -> Relay1/1
  Relay/1 -> m2/1
  Relay1/1 -> m4/1

== system afe_dq_inv_3L_psm/afe_dq_inv_psm_mod1/inverter/inverter/sv_pwm/modulator1/PWM generator v/modulator_p1 ==
  tr : Inport
  m_index : Inport  Port=2
  Constant : Constant  Value=dead_time*f
  Constant1 : Constant  Value=polarity
  Data Type Conversion1 : DataTypeConversion  OutDataTypeStr=double
  Data Type Conversion2 : DataTypeConversion  OutDataTypeStr=double
  Hit Crossing : HitCross  ShowOutputPort=off
  Hit Crossing1 : HitCross  ShowOutputPort=off
  Relational Operator1 : RelationalOperator  Operator=<  InputSameDT=off
  Relational Operator2 : RelationalOperator  Operator=<  InputSameDT=off
  Relay : Relay  OnSwitchValue=2*eps  OnOutputValue=pos_cmd_gate  OffOutputValue=neg_cmd_gate
  Relay1 : Relay  OnOutputValue=pos_cmd_gate  OffOutputValue=neg_cmd_gate
  Saturation1 : Saturate  UpperLimit=m_up  LowerLimit=0
  Sum : Sum  Inputs=|++  SaturateOnIntegerOverflow=on
  Sum1 : Sum  Inputs=-+|  SaturateOnIntegerOverflow=on
  Switch : Switch  Criteria=u2 > Threshold  SaturateOnIntegerOverflow=off  InputSameDT=off
  Switch1 : Switch  Criteria=u2 > Threshold  SaturateOnIntegerOverflow=off  InputSameDT=off
  m1 : Outport
  m3 : Outport  Port=2
  wires:
  Relay1/1 -> m3/1
  Relay/1 -> m1/1
  Switch1/1 -> Relay1/1
  tr/1 -> Relational Operator1/2, Relational Operator2/1
  Sum/1 -> Relational Operator1/1
  Constant/1 -> Sum1/1, Sum/2
  Switch/1 -> Relay/1
  Data Type Conversion2/1 -> Hit Crossing1/1, Switch1/3, Switch/1
  Constant1/1 -> Switch/2, Switch1/2
  Saturation1/1 -> Sum1/2, Sum/1
  Sum1/1 -> Relational Operator2/2
  Data Type Conversion1/1 -> Switch1/1, Switch/3, Hit Crossing/1
  Relational Operator1/1 -> Data Type Conversion1/1
  Relational Operator2/1 -> Data Type Conversion2/1
  m_index/1 -> Saturation1/1

== system afe_dq_inv_3L_psm/afe_dq_inv_psm_mod1/inverter/inverter/sv_pwm/modulator1/PWM generator w/carry_p ==
  phase : Inport
  Clock : Clock
  Constant2 : Constant  Value=1/f
  Constant4 : Constant
  Gain4 : Gain  Gain=1/2
  Gain5 : Gain  Gain=1/(pi/2)
  MATLAB Function : MATLAB Function  TreatAsAtomicUnit=on
  Sum3 : Sum  Inputs=|++
  trp : Outport
  wires:
  Gain5/1 -> Sum3/1
  Gain4/1 -> trp/1
  Constant2/1 -> MATLAB Function/3(period)
  Sum3/1 -> Gain4/1
  MATLAB Function/1(y) -> Gain5/1
  Constant4/1 -> Sum3/2
  Clock/1 -> MATLAB Function/1(t)
  phase/1 -> MATLAB Function/2(phase)

== system afe_dq_inv_3L_psm/afe_dq_inv_psm_mod1/inverter/inverter/sv_pwm/modulator1/PWM generator w/modulator_n1 ==
  tr : Inport
  m_index : Inport  Port=2
  Constant : Constant  Value=dead_time*f
  Constant1 : Constant  Value=polarity
  Constant2 : Constant
  Data Type Conversion1 : DataTypeConversion  OutDataTypeStr=double
  Data Type Conversion2 : DataTypeConversion  OutDataTypeStr=double
  Hit Crossing : HitCross  ShowOutputPort=off
  Hit Crossing1 : HitCross  ShowOutputPort=off
  Relational Operator1 : RelationalOperator  Operator=<  InputSameDT=off
  Relational Operator2 : RelationalOperator  Operator=<=  InputSameDT=off
  Relay : Relay  OnOutputValue=pos_cmd_gate  OffOutputValue=neg_cmd_gate
  Relay1 : Relay  OnOutputValue=pos_cmd_gate  OffOutputValue=neg_cmd_gate
  Saturation1 : Saturate  UpperLimit=0  LowerLimit=m_low
  Sum : Sum  Inputs=|++  SaturateOnIntegerOverflow=on
  Sum1 : Sum  Inputs=-+|  SaturateOnIntegerOverflow=on
  Sum2 : Sum  Inputs=++|  SaturateOnIntegerOverflow=on
  Switch : Switch  Criteria=u2 > Threshold  SaturateOnIntegerOverflow=off  InputSameDT=off
  Switch1 : Switch  Criteria=u2 > Threshold  SaturateOnIntegerOverflow=off  InputSameDT=off
  m2 : Outport
  m4 : Outport  Port=2
  wires:
  Relay1/1 -> m4/1
  Relay/1 -> m2/1
  Switch1/1 -> Relay1/1
  tr/1 -> Relational Operator1/2, Relational Operator2/1
  Sum/1 -> Relational Operator1/1
  Constant/1 -> Sum1/1, Sum/2
  Switch/1 -> Relay/1
  Data Type Conversion2/1 -> Hit Crossing1/1, Switch1/3, Switch/1
  Constant1/1 -> Switch/2, Switch1/2
  Sum1/1 -> Relational Operator2/2
  Data Type Conversion1/1 -> Switch1/1, Switch/3, Hit Crossing/1
  Relational Operator1/1 -> Data Type Conversion1/1
  Relational Operator2/1 -> Data Type Conversion2/1
  m_index/1 -> Saturation1/1
  Saturation1/1 -> Sum2/2
  Sum2/1 -> Sum1/2, Sum/1
  Constant2/1 -> Sum2/1

== system afe_dq_inv_3L_psm/afe_dq_inv_psm_mod1/inverter/inverter/sv_pwm/modulator1/PWM generator w/modulator_p1 ==
  tr : Inport
  m_index : Inport  Port=2
  Constant : Constant  Value=dead_time*f
  Constant1 : Constant  Value=polarity
  Data Type Conversion1 : DataTypeConversion  OutDataTypeStr=double
  Data Type Conversion2 : DataTypeConversion  OutDataTypeStr=double
  Hit Crossing : HitCross  ShowOutputPort=off
  Hit Crossing1 : HitCross  ShowOutputPort=off
  Relational Operator1 : RelationalOperator  Operator=<  InputSameDT=off
  Relational Operator2 : RelationalOperator  Operator=<  InputSameDT=off
  Relay : Relay  OnSwitchValue=2*eps  OnOutputValue=pos_cmd_gate  OffOutputValue=neg_cmd_gate
  Relay1 : Relay  OnOutputValue=pos_cmd_gate  OffOutputValue=neg_cmd_gate
  Saturation1 : Saturate  UpperLimit=m_up  LowerLimit=0
  Sum : Sum  Inputs=|++  SaturateOnIntegerOverflow=on
  Sum1 : Sum  Inputs=-+|  SaturateOnIntegerOverflow=on
  Switch : Switch  Criteria=u2 > Threshold  SaturateOnIntegerOverflow=off  InputSameDT=off
  Switch1 : Switch  Criteria=u2 > Threshold  SaturateOnIntegerOverflow=off  InputSameDT=off
  m1 : Outport
  m3 : Outport  Port=2
  wires:
  m_index/1 -> Saturation1/1
  Relational Operator2/1 -> Data Type Conversion2/1
  Relational Operator1/1 -> Data Type Conversion1/1
  Data Type Conversion1/1 -> Hit Crossing/1, Switch/3, Switch1/1
  Sum1/1 -> Relational Operator2/2
  Saturation1/1 -> Sum/1, Sum1/2
  Constant1/1 -> Switch1/2, Switch/2
  Data Type Conversion2/1 -> Switch/1, Switch1/3, Hit Crossing1/1
  Switch/1 -> Relay/1
  Constant/1 -> Sum/2, Sum1/1
  Sum/1 -> Relational Operator1/1
  tr/1 -> Relational Operator2/1, Relational Operator1/2
  Switch1/1 -> Relay1/1
  Relay/1 -> m1/1
  Relay1/1 -> m3/1

== system afe_dq_inv_3L_psm/afe_dq_inv_psm_mod1/inverter_control/current_ctrl/bemf_observer/phase_fault/hold_phase_for_delta_time/Enabled Subsystem ==
  theta_pmsm : Inport
  Enable : EnablePort
  theta : Outport
  wires:
  theta_pmsm/1 -> theta/1

== system afe_dq_inv_3L_psm/afe_dq_inv_psm_mod1/inverter_control/current_ctrl/bemf_observer/phase_fault/loss_phase/Enabled Subsystem ==
  theta_pmsm : Inport
  Enable : EnablePort
  theta : Outport
  wires:
  theta_pmsm/1 -> theta/1

== system afe_dq_inv_3L_psm/afe_dq_inv_psm_mod1/inverter_control/current_ctrl/current_ctrl/dq_pi_with_vector_antiwindup/dq_vector_pi/bounder1 ==
  md : Inport
  m_1 : Inport  Port=2
  m : Inport  Port=3
  Constant : Constant
  Constant1 : Constant  Value=0
  Divide : Product
  Switch : Switch  Threshold=1  SaturateOnIntegerOverflow=off  InputSameDT=off
  Switch1 : Switch  Threshold=1  SaturateOnIntegerOverflow=off  InputSameDT=off
  md_sat : Outport  VectorParamsAs1DForOutWhenUnconnected=off
  clip : Outport  Port=2  VectorParamsAs1DForOutWhenUnconnected=off
  wires:
  md/1 -> Switch1/3, Divide/2
  m_1/1 -> Divide/1
  Divide/1 -> Switch1/1
  Switch1/1 -> md_sat/1
  Switch/1 -> clip/1
  m/1 -> Switch1/2, Switch/2
  Constant/1 -> Switch/1
  Constant1/1 -> Switch/3

== system afe_dq_inv_3L_psm/afe_dq_inv_psm_mod1/inverter_control/current_ctrl/current_ctrl/dq_pi_with_vector_antiwindup/dq_vector_pi/bounder2 ==
  m : Inport
  m_1 : Inport  Port=2
  mq : Inport  Port=3
  Constant : Constant
  Constant1 : Constant  Value=0
  Divide : Product
  Switch : Switch  Threshold=1  SaturateOnIntegerOverflow=off  InputSameDT=off
  Switch1 : Switch  Threshold=1  SaturateOnIntegerOverflow=off  InputSameDT=off
  mq_sat : Outport  VectorParamsAs1DForOutWhenUnconnected=off
  clip : Outport  Port=2  VectorParamsAs1DForOutWhenUnconnected=off
  wires:
  Constant1/1 -> Switch/3
  Constant/1 -> Switch/1
  m/1 -> Switch1/2, Switch/2
  Switch/1 -> clip/1
  Switch1/1 -> mq_sat/1
  Divide/1 -> Switch1/1
  m_1/1 -> Divide/1
  mq/1 -> Divide/2, Switch1/3

== system afe_dq_inv_3L_psm/afe_dq_inv_psm_mod1/inverter_control/current_ctrl/current_ctrl/dq_pi_with_vector_antiwindup/dq_vector_pi/pi_d ==
  id_tilde : Inport
  clip : Inport  Port=2
  1/Ti : Gain  Gain=kp_i  SaturateOnIntegerOverflow=on  OutDataTypeStr=Inherit: Same as input  ParamDataTypeStr=Inherit: Same as input
  Constant : Constant  Value=0
  Sum2 : Sum  Inputs=+-  SaturateOnIntegerOverflow=on
  Sum4 : Sum  SaturateOnIntegerOverflow=on
  Sum5 : Sum  SaturateOnIntegerOverflow=on
  Switch1 : Switch  Threshold=0.5  SaturateOnIntegerOverflow=off  InputSameDT=off
  Switch2 : Switch  Threshold=0.5  SaturateOnIntegerOverflow=off  InputSameDT=off
  Unit Delay1 : UnitDelay  SampleTime=ts_inv  HasFrameUpgradeWarning=on
  Unit Delay2 : UnitDelay  SampleTime=ts_inv  HasFrameUpgradeWarning=on
  kp1 : Gain  Gain=CTRPIFF_CLIP_RELEASE*ts_inv  SaturateOnIntegerOverflow=on  OutDataTypeStr=Inherit: Same as input  ParamDataTypeStr=Inherit: Same as input
  kp2 : Gain  Gain=ki_i*ts_inv  SaturateOnIntegerOverflow=on  OutDataTypeStr=Inherit: Same as input  ParamDataTypeStr=Inherit: Same as input
  ud_out : Outport  VectorParamsAs1DForOutWhenUnconnected=off
  wires:
  id_tilde/1 -> kp2/1, 1/Ti/1
  Sum5/1 -> ud_out/1
  Switch1/1 -> Unit Delay2/1
  Sum4/1 -> Sum5/2, Switch1/3
  kp1/1 -> Sum2/2
  Sum2/1 -> Switch1/1
  Unit Delay2/1 -> Sum4/2, kp1/1, Sum2/1
  1/Ti/1 -> Sum5/1
  Switch2/1 -> Sum4/1
  kp2/1 -> Switch2/3
  clip/1 -> Unit Delay1/1
  [clip] -> Switch2/2
  [clip] -> Switch1/2
  Constant/1 -> Switch2/1
  Unit Delay1/1 -> [clip]

== system afe_dq_inv_3L_psm/afe_dq_inv_psm_mod1/inverter_control/current_ctrl/current_ctrl/dq_pi_with_vector_antiwindup/dq_vector_pi/pi_q ==
  iq_tilde : Inport
  clip : Inport  Port=2
  1/Ti : Gain  Gain=kp_i  SaturateOnIntegerOverflow=on  OutDataTypeStr=Inherit: Same as input  ParamDataTypeStr=Inherit: Same as input
  Constant : Constant  Value=0
  Sum2 : Sum  Inputs=+-  SaturateOnIntegerOverflow=on
  Sum4 : Sum  SaturateOnIntegerOverflow=on
  Sum5 : Sum  SaturateOnIntegerOverflow=on
  Switch1 : Switch  Threshold=0.5  SaturateOnIntegerOverflow=off  InputSameDT=off
  Switch2 : Switch  Threshold=0.5  SaturateOnIntegerOverflow=off  InputSameDT=off
  Unit Delay1 : UnitDelay  SampleTime=ts_inv  HasFrameUpgradeWarning=on
  Unit Delay2 : UnitDelay  SampleTime=ts_inv  HasFrameUpgradeWarning=on
  kp1 : Gain  Gain=CTRPIFF_CLIP_RELEASE*ts_inv  SaturateOnIntegerOverflow=on  OutDataTypeStr=Inherit: Same as input  ParamDataTypeStr=Inherit: Same as input
  kp2 : Gain  Gain=ki_i*ts_inv  SaturateOnIntegerOverflow=on  OutDataTypeStr=Inherit: Same as input  ParamDataTypeStr=Inherit: Same as input
  Vqs_out : Outport  VectorParamsAs1DForOutWhenUnconnected=off
  wires:
  Constant/1 -> Switch2/1
  [clip] -> Switch1/2
  [clip] -> Switch2/2
  clip/1 -> Unit Delay1/1
  kp2/1 -> Switch2/3
  Switch2/1 -> Sum4/1
  1/Ti/1 -> Sum5/1
  Unit Delay2/1 -> Sum2/1, kp1/1, Sum4/2
  Sum2/1 -> Switch1/1
  kp1/1 -> Sum2/2
  Sum4/1 -> Sum5/2, Switch1/3
  Switch1/1 -> Unit Delay2/1
  iq_tilde/1 -> 1/Ti/1, kp2/1
  Unit Delay1/1 -> [clip]
  Sum5/1 -> Vqs_out/1

== system afe_dq_inv_3L_psm/afe_dq_inv_psm_mod1/inverter_control/current_ctrl/current_ctrl/dq_pi_with_vector_antiwindup/dq_vector_pi/switch ==
  clip 1 : Inport
  clip 2 : Inport  Port=2
  Constant4 : Constant
  Constant5 : Constant  Value=0
  Sum1 : Sum  SaturateOnIntegerOverflow=on
  Switch : Switch  Threshold=0.5  SaturateOnIntegerOverflow=off  InputSameDT=off
  clip : Outport  VectorParamsAs1DForOutWhenUnconnected=off
  wires:
  Constant5/1 -> Switch/3
  Switch/1 -> clip/1
  Constant4/1 -> Switch/1
  Sum1/1 -> Switch/2
  clip 1/1 -> Sum1/1
  clip 2/1 -> Sum1/2

== system afe_dq_inv_3L_psm/afe_dq_inv_psm_mod1/inverter_control/current_ctrl/current_ctrl/dq_pi_with_vector_antiwindup/dq_vector_pi/vector lenght ==
  md : Inport
  mq : Inport  Port=2
  Math Function : Math  Operator=magnitude^2  SignedPower=on
  Math Function1 : Math  Operator=magnitude^2  SignedPower=on
  Math Function2 : Math  Operator=reciprocal  SignedPower=on
  Sqrt : Sqrt
  Sum5 : Sum  SaturateOnIntegerOverflow=on
  m_1 : Outport  VectorParamsAs1DForOutWhenUnconnected=off
  m : Outport  Port=2  VectorParamsAs1DForOutWhenUnconnected=off
  wires:
  Sqrt/1 -> m/1, Math Function2/1
  mq/1 -> Math Function1/1
  Math Function1/1 -> Sum5/2
  Math Function/1 -> Sum5/1
  Sum5/1 -> Sqrt/1
  Math Function2/1 -> m_1/1
  md/1 -> Math Function/1

== system afe_dq_inv_3L_psm/afe_dq_inv_psm_mod1/inverter_control/current_ctrl/current_ctrl/dq_pi_with_vector_antiwindup/dq_vector_pi_ccaller/Reset ==
  Step : Step  Time=0.05  Before=1  After=0  SampleTime=0
  en : Outport
  wires:
  Step/1 -> en/1
